simulink model "pci1756"  (R2016b)
settings: Solver=ode4  StartTime=0.0  StopTime=inf  FixedStep=0.002  RelTol=1e-3  EnableMultiTasking=on
settings Model: SimulationMode=external  Creator=Administrator  LastModifiedBy=Administrator
settings SolverCC: EnableConcurrentExecution=on
settings DataIOCC: SaveFormat=StructureWithTime
settings OptimizationCC: BlockReduction=off  OptimizeBlockIOStorage=off  BufferReuse=off  GlobalBufferReuse=off  ExpressionFolding=off  LocalBlockOutputs=off
settings HardwareCC: ProdBitPerPointer=32  ProdBitPerSizeT=32  ProdBitPerPtrDiffT=32  ProdLargestAtomicFloat=None  ProdWordSize=32  ProdLongLongMode=on  ProdHWDeviceType=Generic->32-bit x86 compatible
settings RTWCC: SystemTargetFile=slrt.tlc  TemplateMakefile=slrt_default_tmf  Description=Simulink Real-Time  RTWCompilerOptimization=on

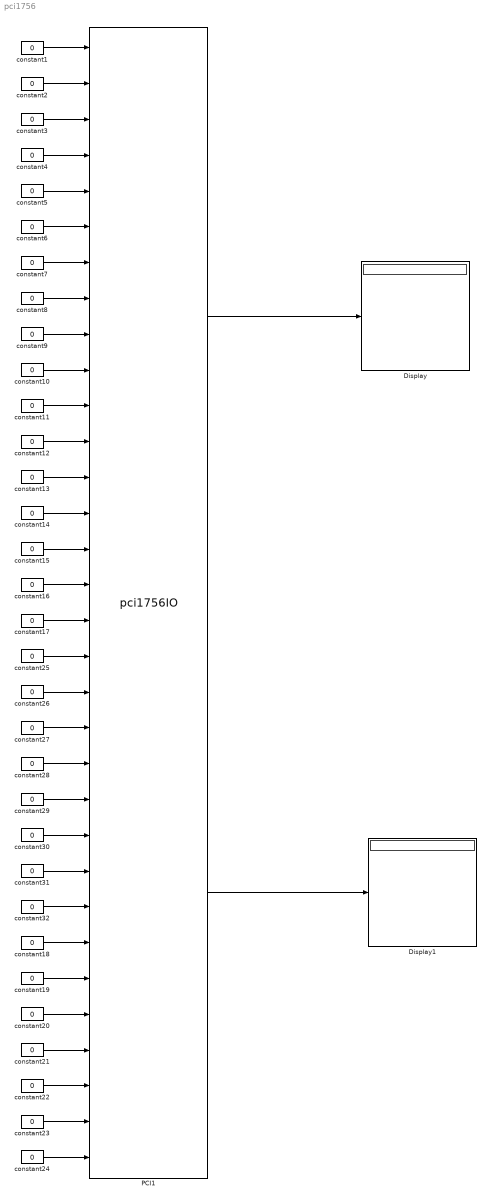
== system pci1756 ==
  Display : Display
  Display1 : Display
  PCI1 : S-Function  FunctionName=pci1756IO  Parameters=[SampleTime SampleOffset], SLOT  SFunctionDeploymentMode=off  EnableBusSupport=off  mask(PCI1756){Sample=0.002, SLOT=[2 11]}
      mask prompts: Sample "Sample time:"
      mask help:
      | PCI-1756
      | Advantech
      | Digital Input&Output
      mask init:
      | SampleTime =0.002; SampleOffset=0;
      mask Display:
      | disp('PCI1756\nDigital output&input\n');
      | port_label('input',1,'DO1');
      | port_label('input',2,'DO2');
      | port_label('input',3,'DO3');
      | port_label('input',4,'DO4');
      | port_label('input',5,'DO5');
      | port_label('input',6,'DO6');
      | port_label('input',7,'DO7');
      | port_label('input',8,'DO8');
      | port_label('input',9,'DO9');
      | port_label('input',10,'DO10');
      | port_label('input',11,'DO11');
      | port_label('input',12,'DO12');
      | port_label('input',13,'DO13');
      | port_label('input',14,'DO14');
      | port_label('input',15,'DO15');
      | port_label('input',16,'DO16');
      | port_label('input',17,'DO17');
      | port_label('input',18,'DO18');
      | port_label('input',19,'DO19');
      | port_label('input',20,'DO20');
      | port_label('input',21,'DO21');
      | port_label('input',22,'DO22');
      | port_label('input',23,'DO23');
      | port_label('input',24,'DO24');
      | port_label('input',25,'DO25');
      | port_label('input',26,'DO26');
      | port_label('input',27,'DO27');
      | port_label('input',28,'DO28');
      | port_label('input',29,'DO29');
      | port_label('input',30,'DO30');
      | port_label('input',31,'DO31');
      | port_label('input',32,'DO32');
      | port_label('output',1,'DI1');
      | port_label('output',2,'DI2');
  constant{1..32} (32 alike) : Constant  Value=0
      settings: OpenFcn=|
      | if get_param(gcb,'value')=='1',
      | set_param(gcb,'value','0');
      | else
      | set_param(gcb,'value','1');end
  wires:
  constant2/1 -> PCI1/2
  constant3/1 -> PCI1/3
  constant4/1 -> PCI1/4
  constant5/1 -> PCI1/5
  constant6/1 -> PCI1/6
  constant7/1 -> PCI1/7
  constant8/1 -> PCI1/8
  constant9/1 -> PCI1/9
  constant10/1 -> PCI1/10
  constant11/1 -> PCI1/11
  constant12/1 -> PCI1/12
  constant13/1 -> PCI1/13
  constant14/1 -> PCI1/14
  constant15/1 -> PCI1/15
  constant16/1 -> PCI1/16
  constant17/1 -> PCI1/17
  constant25/1 -> PCI1/18
  constant26/1 -> PCI1/19
  constant27/1 -> PCI1/20
  constant28/1 -> PCI1/21
  constant29/1 -> PCI1/22
  constant30/1 -> PCI1/23
  constant31/1 -> PCI1/24
  constant32/1 -> PCI1/25
  constant18/1 -> PCI1/26
  constant19/1 -> PCI1/27
  constant20/1 -> PCI1/28
  constant21/1 -> PCI1/29
  constant22/1 -> PCI1/30
  constant23/1 -> PCI1/31
  constant24/1 -> PCI1/32
  PCI1/1 -> Display/1
  constant1/1 -> PCI1/1
  PCI1/2 -> Display1/1
